simulink model "New_Wagon_Position"  (R2016a)
settings: Solver=ode45  StartTime=0.0  StopTime=10.0  RelTol=1e-3
values from neighbouring files (symbols this model uses):
  A = [0,1,0,0;20.9,0,0,0;0,0,0,1;-0.8,0,0,0]    [SSAE_script.m]
  B = [0;-1;0;0.5]    [SSAE_script.m]
  C = [1,0,0,0;0,0,1,0]    [SSAE_script.m]
  K = place(A,B,poles)    [SSAE_script.m]
settings Model: Creator=el12074  LastModifiedBy=dimst
settings DataIOCC: LimitDataPoints=on  SaveFormat=Array
settings DebuggingCC: SolverPrmCheckMsg=warning
settings HardwareCC: ProdBitPerPointer=32  ProdLargestAtomicFloat=None  ProdIntDivRoundTo=Undefined  ProdEndianess=Unspecified  ProdWordSize=32  ProdHWDeviceType=32-bit Generic
settings ModelReferenceCC: PropagateSignalLabelsOutOfModel=off
settings ConfigComp: CovModelRefEnable=Off  CovSFcnEnable=off

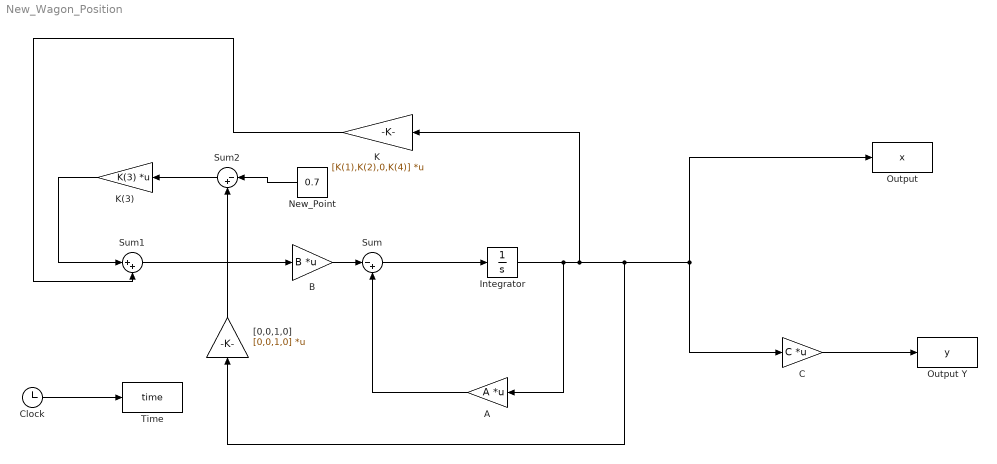
== system New_Wagon_Position ==
  A : Gain  Gain=A  Multiplication=Matrix(K*u)
  B : Gain  Gain=B  Multiplication=Matrix(K*u)
  C : Gain  Gain=C  Multiplication=Matrix(K*u)
  Clock : Clock
  Integrator : Integrator  InitialCondition=[-0.2;-0.06;0.01;0.3]
  New_Point : Constant  Value=0.7
  "Output " : ToWorkspace  VariableName=x  SampleTime=-1
      settings: Save2DSignal=2-D array (concatenate along first dimension)
  Output Y : ToWorkspace  VariableName=y  SampleTime=-1
      settings: Save2DSignal=2-D array (concatenate along first dimension)
  Sum : Sum  Inputs=|-+
  Sum1 : Sum  Inputs=|++
  Sum2 : Sum  Inputs=|-+
  Time : ToWorkspace  VariableName=time  SampleTime=-1
      settings: Save2DSignal=2-D array (concatenate along first dimension)
  "[0,0,1,0]" : Gain  Gain=[0,0,1,0]  Multiplication=Matrix(K*u)
  Κ : Gain  Gain=[K(1),K(2),0,K(4)]  Multiplication=Matrix(K*u)
  Κ(3) : Gain  Gain=K(3)  Multiplication=Matrix(K*u)
  wires:
  B/1 -> Sum/1
  A/1 -> Sum/2
  Sum/1 -> Integrator/1
  C/1 -> Output Y/1
  Clock/1 -> Time/1
  Sum1/1 -> B/1
  New_Point/1 -> Sum2/1
  "[0,0,1,0]"/1 -> Sum2/2
  Sum2/1 -> Κ(3)/1
  Κ(3)/1 -> Sum1/1
  Κ/1 -> Sum1/2
  Integrator/1 -> "Output "/1, C/1, "[0,0,1,0]"/1, Κ/1, A/1
